simulink model "Lab1bPartB3"  (R2023b)
settings: Solver=VariableStepAuto  StartTime=0.0  StopTime=50  RelTol=1e-3
settings Model: Creator=tanvi  LastModifiedBy=tanvi

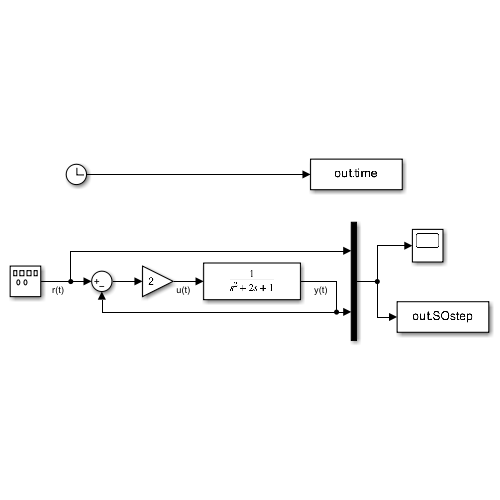
[thumbnail: Simulink's stored preview of the top-level diagram]
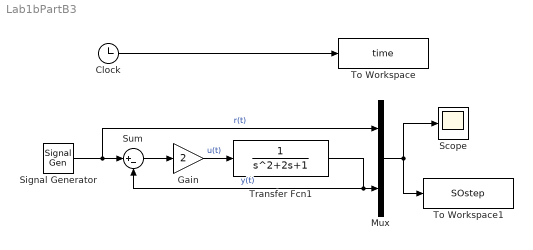
== system Lab1bPartB3 ==
  Clock : Clock
      settings: Decimation=100
  Gain : Gain  Gain=2
  Mux : Mux  Inputs=2
  Scope : Scope
  Signal Generator : SignalGenerator  WaveForm=square  Frequency=0.05
  Sum : Sum  Inputs=|+-
  To Workspace : ToWorkspace  VariableName=time  SampleTime=-1
  To Workspace1 : ToWorkspace  VariableName=SOstep  SampleTime=-1
  Transfer Fcn1 : TransferFcn
  wires:
  Clock/1 -> To Workspace/1
  Mux/1 -> Scope/1, To Workspace1/1
  Gain/1 -> Transfer Fcn1/1  "u(t)"
  Signal Generator/1 -> Mux/1, Sum/1  "r(t)"
  Sum/1 -> Gain/1
  Transfer Fcn1/1 -> Sum/2, Mux/2  "y(t)"
